simulink model "48Vto200V_statespace"  (R2026a)
settings: Solver=VariableStepAuto  StopTime=0.1
settings Model: Creator=riddh  LastModifiedBy=riddh

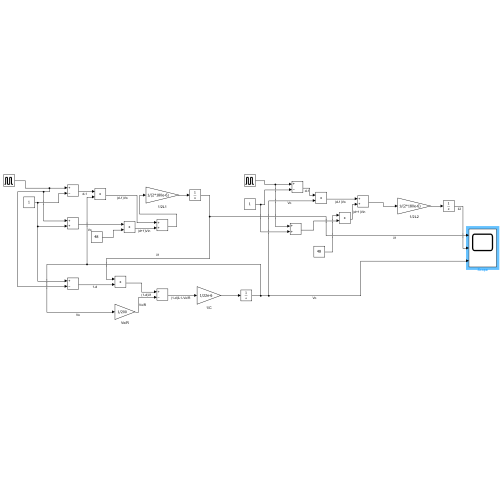
[thumbnail: Simulink's stored preview of the top-level diagram]
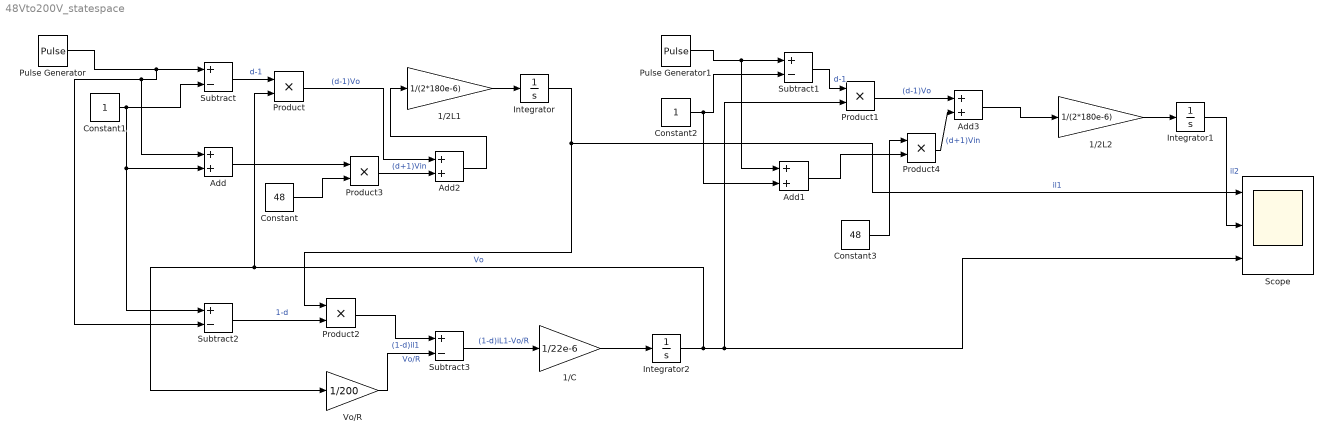
== system 48Vto200V_statespace ==
  1/2L1 : Gain  Gain=1/(2*180e-6)
  1/2L2 : Gain  Gain=1/(2*180e-6)
  1/C : Gain  Gain=1/22e-6
  Add{,1..3} (4 alike) : Sum
  Constant : Constant  Value=48
  Constant1 : Constant
  Constant2 : Constant
  Constant3 : Constant  Value=48
  Integrator : Integrator
  Integrator1 : Integrator
  Integrator2 : Integrator
  Product{,1..4} (5 alike) : Product
  Pulse Generator : DiscretePulseGenerator  PulseType=Time based  Period=1/50e3  PulseWidth=61
  Pulse Generator1 : DiscretePulseGenerator  PulseType=Time based  Period=1/50e3  PulseWidth=61
  Scope : Scope  NumInputPorts=3
      settings: ActiveDisplayYMinimum=-17.518415437833397  ActiveDisplayYMaximum=9.7290722744091731
  Subtract{,1..3} (4 alike) : Sum  Inputs=+-
  Vo/R : Gain  Gain=1/200
  wires:
  Pulse Generator/1 -> Subtract/1, Add/1, Subtract2/2
  Constant1/1 -> Subtract/2, Add/2, Subtract2/1
  Subtract/1 -> Product/1  "d-1"
  Product/1 -> Add2/1  "(d-1)Vo"
  Pulse Generator1/1 -> Add1/1, Subtract1/1
  Constant2/1 -> Add1/2, Subtract1/2
  Subtract1/1 -> Product1/1  "d-1"
  1/2L1/1 -> Integrator/1
  Integrator/1 -> Product2/1, Scope/1  "il1"
  Integrator1/1 -> Scope/2  "il2"
  1/2L2/1 -> Integrator1/1
  Subtract2/1 -> Product2/2  "1-d"
  Product2/1 -> Subtract3/1  "(1-d)il1"
  Vo/R/1 -> Subtract3/2  "Vo/R"
  Subtract3/1 -> 1/C/1  "(1-d)iL1-Vo/R"
  1/C/1 -> Integrator2/1
  Integrator2/1 -> Scope/3, Product1/2, Vo/R/1, Product/2  "Vo"
  Add/1 -> Product3/1
  Constant/1 -> Product3/2
  Product3/1 -> Add2/2  "(d+1)Vin"
  Add2/1 -> 1/2L1/1
  Add1/1 -> Product4/2
  Constant3/1 -> Product4/1
  Product1/1 -> Add3/1  "(d-1)Vo"
  Product4/1 -> Add3/2  "(d+1)Vin"
  Add3/1 -> 1/2L2/1
